simulink model "step4"  (R2018b)
settings: Solver=VariableStepAuto  StartTime=0  StopTime=5000  RelTol=1e-3
values from neighbouring files (symbols this model uses):
  AM = K(i)    [step4part1.m]    (also in step4part2.m = 50; step5part2.m = 50; step5part3.m = 50)
  k = -0.004188    [step4part1.m]    (also in step4part2.m = -457/(300*(tc(i) +73)); step5part1.m = -457/(300*(tc(i)*564 +73)); step5part2.m = -457/(300*(tc(i)*564 +73)); step5part3.m = -457/((k_num(i)./40)*(282 +theta(j))))
  Ts = K(i)    [step3part2.m]    (also in step4part1.m = 10; step4part2.m = 10; step5part2.m = 10; step5part3.m = 10)
libraries: powerlib_meascontrol x1
settings Model: Creator=Asus  LastModifiedBy=Asus
settings OptimizationCC: DefaultParameterBehavior=Inlined  BufferReuse=off
settings DebuggingCC: InitInArrayFormatMsg=none

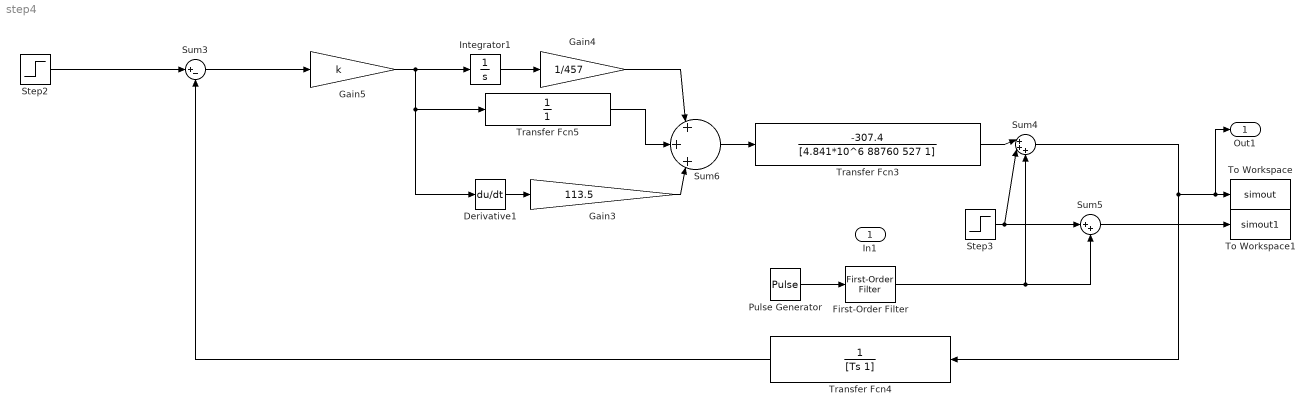
== system step4 ==
  In1 : Inport
  Derivative1 : Derivative
  First-Order Filter : powerlib_meascontrol/Filters/First-Order Filter  FilterType=Lowpass  Tc=50  Ts=0  Initialize=on  Vac_Init=[0, 0, 20]  Vdc_Init=0  PlotResponse=off  FreqRange="[0,  200,  1]"
      settings: SourceProductName=Simscape Power Systems
  Gain3 : Gain  Gain=113.5
  Gain4 : Gain  Gain=1/457
  Gain5 : Gain  Gain=k
  Integrator1 : Integrator
  Pulse Generator : DiscretePulseGenerator  PulseType=Time based  Amplitude=AM  Period=10000  PhaseDelay=4000
  Step2 : Step  After=110  SampleTime=0
  Step3 : Step  After=110  SampleTime=0
  Sum3 : Sum  Inputs=|+-
  Sum4 : Sum  Inputs=|+++
  Sum5 : Sum  Inputs=|++
  Sum6 : Sum  Inputs=|+||+||+|
  To Workspace : ToWorkspace  VariableName=simout  SaveFormat=Timeseries  SampleTime=10
  To Workspace1 : ToWorkspace  VariableName=simout1  SaveFormat=Timeseries  SampleTime=-1
  Transfer Fcn3 : TransferFcn  Numerator=[-307.4]  Denominator=[4.841*10^6 88760 527 1]
  Transfer Fcn4 : TransferFcn  Denominator=[Ts 1]
  Transfer Fcn5 : TransferFcn  Denominator=[1]
  Out1 : Outport
  wires:
  Sum4/1 -> Out1/1, To Workspace/1, Transfer Fcn4/1
  Step2/1 -> Sum3/1
  Transfer Fcn4/1 -> Sum3/2
  Transfer Fcn3/1 -> Sum4/1
  Step3/1 -> Sum5/1, Sum4/2
  Transfer Fcn5/1 -> Sum6/2
  Integrator1/1 -> Gain4/1
  Gain3/1 -> Sum6/3
  Derivative1/1 -> Gain3/1
  Gain5/1 -> Derivative1/1, Transfer Fcn5/1, Integrator1/1
  Gain4/1 -> Sum6/1
  Sum6/1 -> Transfer Fcn3/1
  Sum3/1 -> Gain5/1
  Sum5/1 -> To Workspace1/1
  Pulse Generator/1 -> First-Order Filter/1
  First-Order Filter/1 -> Sum4/3, Sum5/2
